simulink model "alpha147gta"  (R2017b)
settings: Solver=VariableStepAuto  StartTime=0.0  StopTime=10.0  RelTol=1e-3
values from neighbouring files (symbols this model uses):
  EngineRPM = [1000 1500 2000 2500 3000 3500 4000 4500 5000 5500 6000 6500 ... (13 elements, 1x13)]    [alpha147gta.mat]    (also in cruise_control_external.mat; cruise_control_sim.mat)
  EngineTRQ = [200 220 242 258 260 261 268 285 300 296 290 250 ... (13 elements, 1x13)]    [alpha147gta.mat]    (also in cruise_control_external.mat; cruise_control_sim.mat)
  FinalRatio = 3.733    [alpha147gta.mat]    (also in cruise_control_external.mat; cruise_control_sim.mat)
  GearRatio = [3.5 2.235 1.52 1.156 0.971 0.818]    [alpha147gta.mat]    (also in cruise_control_external.mat; cruise_control_sim.mat)
  Kdrag = 0.4238432    [alpha147gta.mat]    (also in cruise_control_external.mat; cruise_control_sim.mat)
  Mass = 1360    [alpha147gta.mat]    (also in cruise_control_external.mat; cruise_control_sim.mat)
  WheelRadius = 0.2992    [alpha147gta.mat]    (also in cruise_control_external.mat; cruise_control_sim.mat)
settings Model: Creator=Rehaan M. Bhimani  LastModifiedBy=Rehaan M. Bhimani

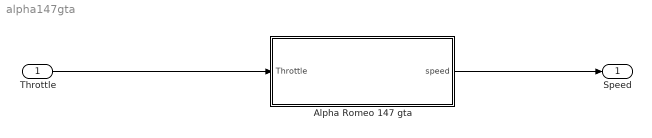
== system alpha147gta ==
  Throttle : Inport
  Alpha Romeo 147 gta : Subsystem
  Speed : Outport
  wires:
  Throttle/1 -> Alpha Romeo 147 gta/1(Throttle)
  Alpha Romeo 147 gta/1(speed) -> Speed/1

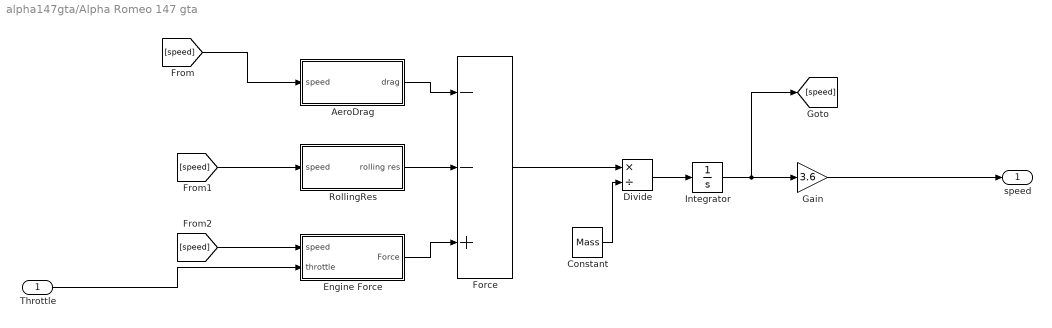
== system alpha147gta/Alpha Romeo 147 gta ==
  Throttle : Inport
  AeroDrag : Subsystem
  Constant : Constant  Value=Mass
  Divide : Product  Inputs=*/
  Engine Force : Subsystem
  Force : Sum  Inputs=--+
  Gain : Gain  Gain=3.6
  Integrator : Integrator
  RollingRes : Subsystem
  speed : Outport
  wires:
  Throttle/1 -> Engine Force/2(throttle)
  [speed] -> Engine Force/1(speed)
  Gain/1 -> speed/1
  Force/1 -> Divide/1
  RollingRes/1(rolling res) -> Force/2
  AeroDrag/1(drag) -> Force/1
  [speed] -> RollingRes/1(speed)
  Engine Force/1(Force) -> Force/3
  Divide/1 -> Integrator/1
  Integrator/1 -> [speed], Gain/1
  Constant/1 -> Divide/2
  [speed] -> AeroDrag/1(speed)

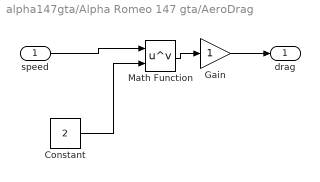
== system alpha147gta/Alpha Romeo 147 gta/AeroDrag ==
  speed : Inport
  Constant : Constant  Value=2
  Gain : Gain
  Math Function : Math  Operator=pow  SaturateOnIntegerOverflow=on
  drag : Outport
  wires:
  Gain/1 -> drag/1
  Math Function/1 -> Gain/1
  Constant/1 -> Math Function/2
  speed/1 -> Math Function/1

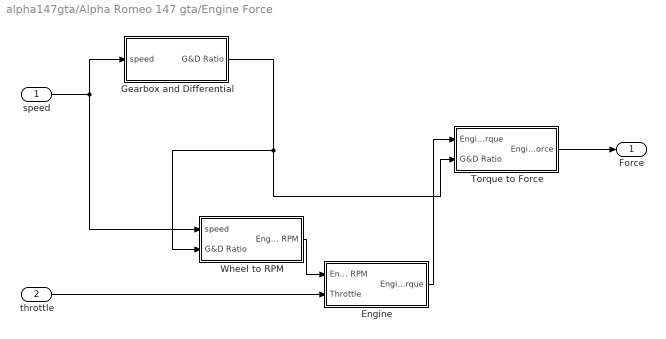
== system alpha147gta/Alpha Romeo 147 gta/Engine Force ==
  speed : Inport
  throttle : Inport  Port=2
  Engine : Subsystem
  Gearbox and Differential : Subsystem
  Torque to Force : Subsystem
  Wheel to RPM : Subsystem
  Force : Outport
  wires:
  speed/1 -> Wheel to RPM/1(speed), Gearbox and Differential/1(speed)
  throttle/1 -> Engine/2(Throttle)
  Gearbox and Differential/1(G&D Ratio) -> Torque to Force/2(G&D Ratio), Wheel to RPM/2(G&D Ratio)
  Wheel to RPM/1(Engine RPM) -> Engine/1("Engine RPM ")
  Engine/1(Engine Torque) -> Torque to Force/1(Engine Torque)
  Torque to Force/1(Engine Force) -> Force/1

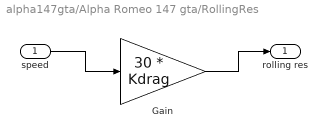
== system alpha147gta/Alpha Romeo 147 gta/RollingRes ==
  speed : Inport
  Gain : Gain  Gain=30 * Kdrag
  rolling res : Outport
  wires:
  speed/1 -> Gain/1
  Gain/1 -> rolling res/1

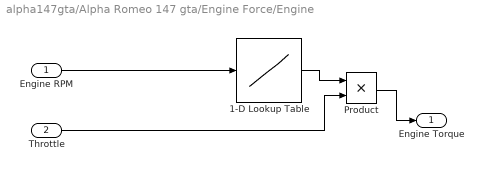
== system alpha147gta/Alpha Romeo 147 gta/Engine Force/Engine ==
  "Engine RPM " : Inport
  Throttle : Inport  Port=2
  1-D Lookup Table : Lookup_n-D  NumberOfTableDimensions=1  BreakpointsForDimension1=EngineRPM  Table=EngineTRQ  InterpMethod=Cubic spline  InternalRulePriority=Speed  RndMeth=Simplest  InputSameDT=on
  Product : Product
  Engine Torque : Outport
  wires:
  "Engine RPM "/1 -> 1-D Lookup Table/1
  1-D Lookup Table/1 -> Product/1
  Throttle/1 -> Product/2
  Product/1 -> Engine Torque/1

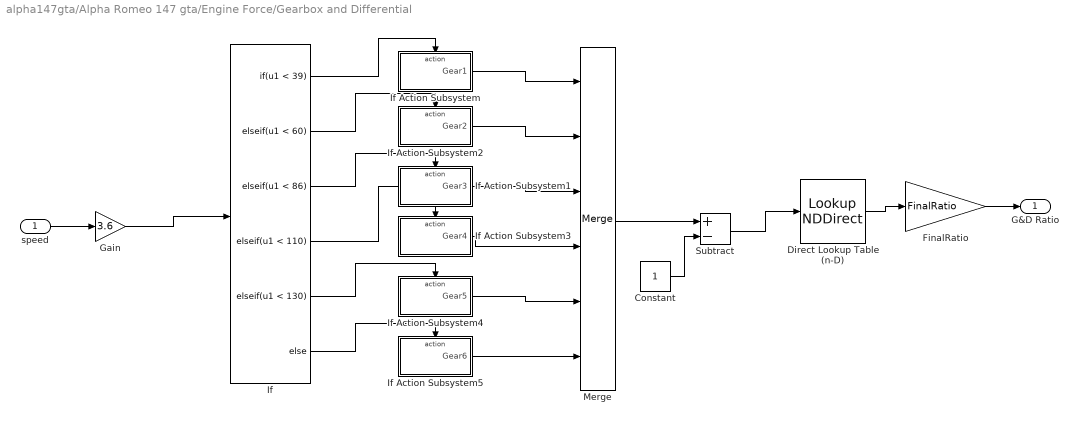
== system alpha147gta/Alpha Romeo 147 gta/Engine Force/Gearbox and Differential ==
  speed : Inport
  Constant : Constant
  Direct Lookup Table (n-D) : LookupNDDirect  NumberOfTableDimensions=1  Table=GearRatio
  FinalRatio : Gain  Gain=FinalRatio
  Gain : Gain  Gain=3.6
  If : If  IfExpression=u1 < 39  ElseIfExpressions=u1 < 60, u1 < 86, u1 < 110, u1 < 130
  If Action Subsystem : Subsystem  TreatAsAtomicUnit=on
  If Action Subsystem1 : Subsystem  TreatAsAtomicUnit=on
  If Action Subsystem2 : Subsystem  TreatAsAtomicUnit=on
  If Action Subsystem3 : Subsystem  TreatAsAtomicUnit=on
  If Action Subsystem4 : Subsystem  TreatAsAtomicUnit=on
  If Action Subsystem5 : Subsystem  TreatAsAtomicUnit=on
  Merge : Merge  Inputs=6
  Subtract : Sum  Inputs=+-
  G&D Ratio : Outport
  wires:
  speed/1 -> Gain/1
  Gain/1 -> If/1
  If/1 -> If Action Subsystem/Action
  If/2 -> If Action Subsystem2/Action
  If/3 -> If Action Subsystem1/Action
  If/4 -> If Action Subsystem3/Action
  If/5 -> If Action Subsystem4/Action
  If/6 -> If Action Subsystem5/Action
  If Action Subsystem/1(Gear1) -> Merge/1
  If Action Subsystem2/1(Gear2) -> Merge/2
  If Action Subsystem1/1("Gear3 ") -> Merge/3
  If Action Subsystem3/1(Gear4) -> Merge/4
  If Action Subsystem4/1(Gear5) -> Merge/5
  If Action Subsystem5/1(Gear6) -> Merge/6
  Merge/1 -> Subtract/1
  Constant/1 -> Subtract/2
  Subtract/1 -> Direct Lookup Table (n-D)/1
  Direct Lookup Table (n-D)/1 -> FinalRatio/1
  FinalRatio/1 -> G&D Ratio/1

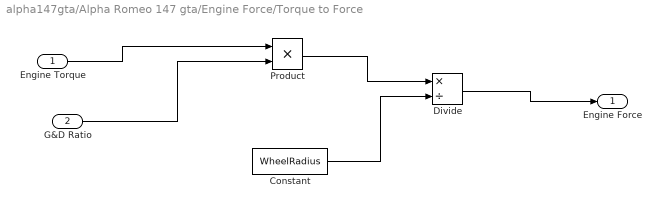
== system alpha147gta/Alpha Romeo 147 gta/Engine Force/Torque to Force ==
  Engine Torque : Inport
  G&D Ratio : Inport  Port=2
  Constant : Constant  Value=WheelRadius
  Divide : Product  Inputs=*/
  Product : Product
  Engine Force : Outport
  wires:
  Constant/1 -> Divide/2
  G&D Ratio/1 -> Product/2
  Engine Torque/1 -> Product/1
  Product/1 -> Divide/1
  Divide/1 -> Engine Force/1

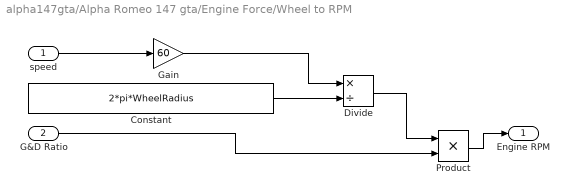
== system alpha147gta/Alpha Romeo 147 gta/Engine Force/Wheel to RPM ==
  speed : Inport
  G&D Ratio : Inport  Port=2
  Constant : Constant  Value=2*pi*WheelRadius
  Divide : Product  Inputs=*/
  Gain : Gain  Gain=60
  Product : Product
  Engine RPM : Outport
  wires:
  speed/1 -> Gain/1
  Gain/1 -> Divide/1
  Constant/1 -> Divide/2
  Divide/1 -> Product/1
  G&D Ratio/1 -> Product/2
  Product/1 -> Engine RPM/1

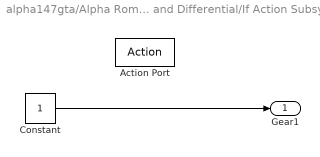
== system alpha147gta/Alpha Romeo 147 gta/Engine Force/Gearbox and Differential/If Action Subsystem ==
  Action Port : ActionPort  ActionType=then
  Constant : Constant
  Gear1 : Outport
  wires:
  Constant/1 -> Gear1/1

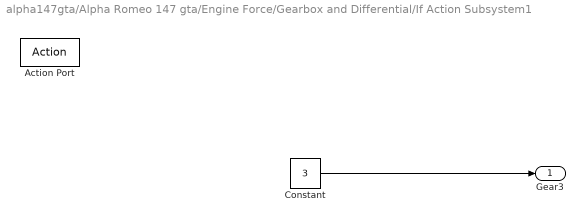
== system alpha147gta/Alpha Romeo 147 gta/Engine Force/Gearbox and Differential/If Action Subsystem1 ==
  Action Port : ActionPort  ActionType=elseif
  Constant : Constant  Value=3
  "Gear3 " : Outport
  wires:
  Constant/1 -> "Gear3 "/1

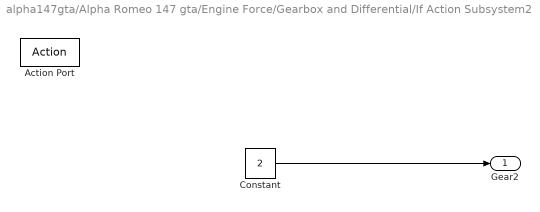
== system alpha147gta/Alpha Romeo 147 gta/Engine Force/Gearbox and Differential/If Action Subsystem2 ==
  Action Port : ActionPort  ActionType=elseif
  Constant : Constant  Value=2
  Gear2 : Outport
  wires:
  Constant/1 -> Gear2/1

== system alpha147gta/Alpha Romeo 147 gta/Engine Force/Gearbox and Differential/If Action Subsystem3 ==
  Action Port : ActionPort  ActionType=elseif
  Constant : Constant  Value=4
  Gear4 : Outport
  wires:
  Constant/1 -> Gear4/1

== system alpha147gta/Alpha Romeo 147 gta/Engine Force/Gearbox and Differential/If Action Subsystem4 ==
  Action Port : ActionPort  ActionType=elseif
  Constant : Constant  Value=5
  Gear5 : Outport
  wires:
  Constant/1 -> Gear5/1

== system alpha147gta/Alpha Romeo 147 gta/Engine Force/Gearbox and Differential/If Action Subsystem5 ==
  Action Port : ActionPort  ActionType=else
  Constant : Constant  Value=6
  Gear6 : Outport
  wires:
  Constant/1 -> Gear6/1
